simulink model "Xl_ch16_LPF_int_v5"  (Simulink 7.5)
settings: Solver=VariableStepDiscrete  StartTime=0.0  StopTime=0.001  RelTol=1e-3
values from neighbouring files (symbols this model uses):
  a2a = zeros(nFc, length(Hd.sosMatrix(:,5)))    [iirButter_SOS_init_v2.m]    (also in iirButter_SOS_init_v2_8pole.m)
  a3a = zeros(nFc, length(Hd.sosMatrix(:,6)))    [iirButter_SOS_init_v2.m]    (also in iirButter_SOS_init_v2_8pole.m)
  dt = 1/Fsim    (= 2.56e-06)    [iirButter_SOS_init_v2.m]    (also in iirButter_SOS_init_v2_8pole.m)
  Fc_min = 10    [iirButter_SOS_init_v2.m]    (also in iirButter_SOS_init_v2_8pole.m)
  ga = zeros(nFc, length(Hd.ScaleValues))    [iirButter_SOS_init_v2.m]    (also in iirButter_SOS_init_v2_8pole.m = zeros(nFc, length(Hd.ScaleValues(1:end-1))))
  rFc = (Fc_max/Fc_min)^(1/(nFc - 1))    (= 1.70532863139)    [iirButter_SOS_init_v2.m]    (also in iirButter_SOS_init_v2_8pole.m)
  Sra = 2^34|.02  |.027 |.027 |<.038| 1e-6|<2e-6|<2e-6|<2e-6|<2e-6| 8e-6|    [iirButter_SOS_init_v2.m]    (also in iirButter_SOS_init_v2_8pole.m)
  Srm = 2^34|     |     |     |     |     |     |     |     |     |  to |    [iirButter_SOS_init_v2.m]    (also in iirButter_SOS_init_v2_8pole.m)
libraries: xbsIndex_r4 x581, dspsrcs4 x16, simulink x8
(part 2 of 4)

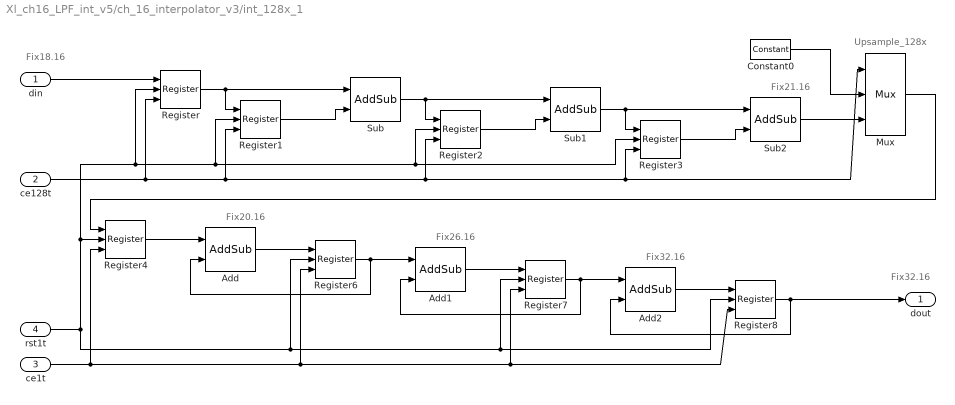
== system Xl_ch16_LPF_int_v5/ch_16_interpolator_v3/int_128x_1 ==
  note: Fix32.16
  note: Fix26.16
  note: Fix20.16
  note: Fix21.16
  note: Upsample_128x
  note: Fix32.16
  note: Fix18.16
  din : Inport
  ce128t : Inport  Port=2
  ce1t : Inport  Port=3
  rst1t : Inport  Port=4
  Add : xbsIndex_r4/AddSub  mode=Addition  use_carryin=off  use_carryout=off  en=off  latency=0  precision=User Defined  arith_type="Signed  (2's comp)"  n_bits=20  bin_pt=16  quantization=Truncate  overflow=Wrap  dbl_ovrd=off  use_behavioral_HDL=off  hw_selection=Fabric  pipelined=off  block_type=addsub
      settings: block_version=12.2
  Add1 : xbsIndex_r4/AddSub  mode=Addition  use_carryin=off  use_carryout=off  en=off  latency=0  precision=User Defined  arith_type="Signed  (2's comp)"  n_bits=26  bin_pt=16  quantization=Truncate  overflow=Wrap  dbl_ovrd=off  use_behavioral_HDL=off  hw_selection=Fabric  pipelined=off  block_type=addsub
      settings: block_version=12.2
  Add2 : xbsIndex_r4/AddSub  mode=Addition  use_carryin=off  use_carryout=off  en=off  latency=0  precision=User Defined  arith_type="Signed  (2's comp)"  n_bits=32  bin_pt=16  quantization=Truncate  overflow=Wrap  dbl_ovrd=off  use_behavioral_HDL=off  hw_selection=Fabric  pipelined=off  block_type=addsub
      settings: block_version=12.2
  Constant0 : xbsIndex_r4/Constant  arith_type=Signed (2's comp)  const=0  n_bits=21  bin_pt=16  explicit_period=off  period=1  equ=P=C  opselect=C  inp2=PCIN>>17  opr=+  inp1=P  carry=CIN  dbl_ovrd=off  block_type=constant
      settings: block_version=12.2
  Mux : xbsIndex_r4/Mux  inputs=2  en=off  latency=0  precision=Full  arith_type=Unsigned  n_bits=16  bin_pt=14  quantization=Truncate  overflow=Wrap  dbl_ovrd=off  block_type=mux
      settings: block_version=12.2
  Register{,1..4,6..8} (8 alike) : xbsIndex_r4/Register  init=0  rst=on  en=on  dbl_ovrd=off  block_type=register
      settings: block_version=12.2
  Sub : xbsIndex_r4/AddSub  mode=Subtraction  use_carryin=off  use_carryout=off  en=off  latency=0  precision=Full  arith_type=Unsigned  n_bits=16  bin_pt=14  quantization=Truncate  overflow=Wrap  dbl_ovrd=off  use_behavioral_HDL=off  hw_selection=Fabric  pipelined=off  block_type=addsub
      settings: block_version=12.2
  Sub1 : xbsIndex_r4/AddSub  mode=Subtraction  use_carryin=off  use_carryout=off  en=off  latency=0  precision=Full  arith_type=Unsigned  n_bits=16  bin_pt=14  quantization=Truncate  overflow=Wrap  dbl_ovrd=off  use_behavioral_HDL=off  hw_selection=Fabric  pipelined=off  block_type=addsub
      settings: block_version=12.2
  Sub2 : xbsIndex_r4/AddSub  mode=Subtraction  use_carryin=off  use_carryout=off  en=off  latency=0  precision=Full  arith_type=Unsigned  n_bits=16  bin_pt=14  quantization=Truncate  overflow=Wrap  dbl_ovrd=off  use_behavioral_HDL=off  hw_selection=Fabric  pipelined=off  block_type=addsub
      settings: block_version=12.2
  dout : Outport
  wires:
  rst1t/1 -> Register/2, Register1/2, Register2/2, Register3/2, Register4/2, Register6/2, Register7/2, Register8/2
  ce1t/1 -> Register4/3, Register6/3, Register8/3, Register7/3
  ce128t/1 -> Register/3, Register1/3, Mux/1, Register3/3, Register2/3
  Register8/1 -> dout/1, Add2/2
  Register7/1 -> Add2/1, Add1/2
  Register6/1 -> Add1/1, Add/2
  Constant0/1 -> Mux/2
  Add2/1 -> Register8/1
  Add1/1 -> Register7/1
  Add/1 -> Register6/1
  Register4/1 -> Add/1
  Mux/1 -> Register4/1
  din/1 -> Register/1
  Sub2/1 -> Mux/3
  Register3/1 -> Sub2/2
  Sub1/1 -> Register3/1, Sub2/1
  Register2/1 -> Sub1/2
  Sub/1 -> Register2/1, Sub1/1
  Register1/1 -> Sub/2
  Register/1 -> Register1/1, Sub/1

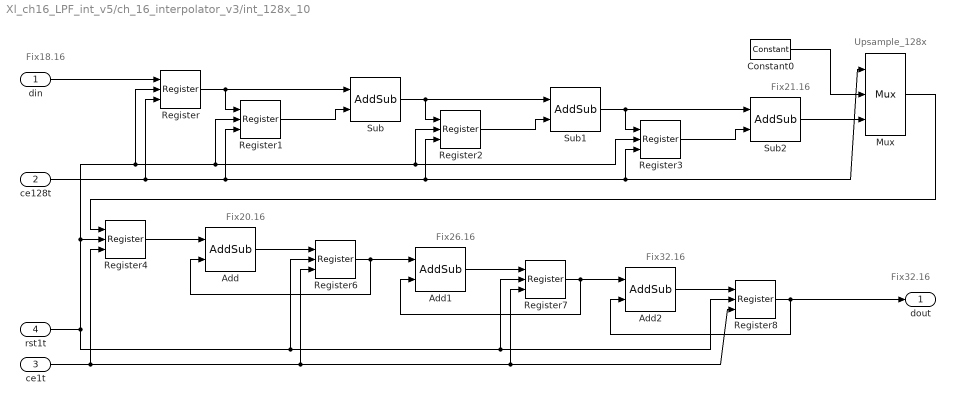
== system Xl_ch16_LPF_int_v5/ch_16_interpolator_v3/int_128x_10 ==
  note: Fix32.16
  note: Fix26.16
  note: Fix20.16
  note: Fix21.16
  note: Upsample_128x
  note: Fix32.16
  note: Fix18.16
  din : Inport
  ce128t : Inport  Port=2
  ce1t : Inport  Port=3
  rst1t : Inport  Port=4
  Add : xbsIndex_r4/AddSub  mode=Addition  use_carryin=off  use_carryout=off  en=off  latency=0  precision=User Defined  arith_type="Signed  (2's comp)"  n_bits=20  bin_pt=16  quantization=Truncate  overflow=Wrap  dbl_ovrd=off  use_behavioral_HDL=off  hw_selection=Fabric  pipelined=off  block_type=addsub
      settings: block_version=12.2
  Add1 : xbsIndex_r4/AddSub  mode=Addition  use_carryin=off  use_carryout=off  en=off  latency=0  precision=User Defined  arith_type="Signed  (2's comp)"  n_bits=26  bin_pt=16  quantization=Truncate  overflow=Wrap  dbl_ovrd=off  use_behavioral_HDL=off  hw_selection=Fabric  pipelined=off  block_type=addsub
      settings: block_version=12.2
  Add2 : xbsIndex_r4/AddSub  mode=Addition  use_carryin=off  use_carryout=off  en=off  latency=0  precision=User Defined  arith_type="Signed  (2's comp)"  n_bits=32  bin_pt=16  quantization=Truncate  overflow=Wrap  dbl_ovrd=off  use_behavioral_HDL=off  hw_selection=Fabric  pipelined=off  block_type=addsub
      settings: block_version=12.2
  Constant0 : xbsIndex_r4/Constant  arith_type=Signed (2's comp)  const=0  n_bits=21  bin_pt=16  explicit_period=off  period=1  equ=P=C  opselect=C  inp2=PCIN>>17  opr=+  inp1=P  carry=CIN  dbl_ovrd=off  block_type=constant
      settings: block_version=12.2
  Mux : xbsIndex_r4/Mux  inputs=2  en=off  latency=0  precision=Full  arith_type=Unsigned  n_bits=16  bin_pt=14  quantization=Truncate  overflow=Wrap  dbl_ovrd=off  block_type=mux
      settings: block_version=12.2
  Register{,1..4,6..8} (8 alike) : xbsIndex_r4/Register  init=0  rst=on  en=on  dbl_ovrd=off  block_type=register
      settings: block_version=12.2
  Sub : xbsIndex_r4/AddSub  mode=Subtraction  use_carryin=off  use_carryout=off  en=off  latency=0  precision=Full  arith_type=Unsigned  n_bits=16  bin_pt=14  quantization=Truncate  overflow=Wrap  dbl_ovrd=off  use_behavioral_HDL=off  hw_selection=Fabric  pipelined=off  block_type=addsub
      settings: block_version=12.2
  Sub1 : xbsIndex_r4/AddSub  mode=Subtraction  use_carryin=off  use_carryout=off  en=off  latency=0  precision=Full  arith_type=Unsigned  n_bits=16  bin_pt=14  quantization=Truncate  overflow=Wrap  dbl_ovrd=off  use_behavioral_HDL=off  hw_selection=Fabric  pipelined=off  block_type=addsub
      settings: block_version=12.2
  Sub2 : xbsIndex_r4/AddSub  mode=Subtraction  use_carryin=off  use_carryout=off  en=off  latency=0  precision=Full  arith_type=Unsigned  n_bits=16  bin_pt=14  quantization=Truncate  overflow=Wrap  dbl_ovrd=off  use_behavioral_HDL=off  hw_selection=Fabric  pipelined=off  block_type=addsub
      settings: block_version=12.2
  dout : Outport
  wires:
  rst1t/1 -> Register/2, Register1/2, Register2/2, Register3/2, Register4/2, Register6/2, Register7/2, Register8/2
  ce1t/1 -> Register4/3, Register6/3, Register8/3, Register7/3
  ce128t/1 -> Register/3, Register1/3, Mux/1, Register3/3, Register2/3
  Register8/1 -> dout/1, Add2/2
  Register7/1 -> Add2/1, Add1/2
  Register6/1 -> Add1/1, Add/2
  Constant0/1 -> Mux/2
  Add2/1 -> Register8/1
  Add1/1 -> Register7/1
  Add/1 -> Register6/1
  Register4/1 -> Add/1
  Mux/1 -> Register4/1
  din/1 -> Register/1
  Sub2/1 -> Mux/3
  Register3/1 -> Sub2/2
  Sub1/1 -> Register3/1, Sub2/1
  Register2/1 -> Sub1/2
  Sub/1 -> Register2/1, Sub1/1
  Register1/1 -> Sub/2
  Register/1 -> Register1/1, Sub/1

== system Xl_ch16_LPF_int_v5/ch_16_interpolator_v3/int_128x_11 ==
  note: Fix18.16
  note: Fix32.16
  note: Upsample_128x
  note: Fix21.16
  note: Fix20.16
  note: Fix26.16
  note: Fix32.16
  din : Inport
  ce128t : Inport  Port=2
  ce1t : Inport  Port=3
  rst1t : Inport  Port=4
  Add : xbsIndex_r4/AddSub  mode=Addition  use_carryin=off  use_carryout=off  en=off  latency=0  precision=User Defined  arith_type="Signed  (2's comp)"  n_bits=20  bin_pt=16  quantization=Truncate  overflow=Wrap  dbl_ovrd=off  use_behavioral_HDL=off  hw_selection=Fabric  pipelined=off  block_type=addsub
      settings: block_version=12.2
  Add1 : xbsIndex_r4/AddSub  mode=Addition  use_carryin=off  use_carryout=off  en=off  latency=0  precision=User Defined  arith_type="Signed  (2's comp)"  n_bits=26  bin_pt=16  quantization=Truncate  overflow=Wrap  dbl_ovrd=off  use_behavioral_HDL=off  hw_selection=Fabric  pipelined=off  block_type=addsub
      settings: block_version=12.2
  Add2 : xbsIndex_r4/AddSub  mode=Addition  use_carryin=off  use_carryout=off  en=off  latency=0  precision=User Defined  arith_type="Signed  (2's comp)"  n_bits=32  bin_pt=16  quantization=Truncate  overflow=Wrap  dbl_ovrd=off  use_behavioral_HDL=off  hw_selection=Fabric  pipelined=off  block_type=addsub
      settings: block_version=12.2
  Constant0 : xbsIndex_r4/Constant  arith_type=Signed (2's comp)  const=0  n_bits=21  bin_pt=16  explicit_period=off  period=1  equ=P=C  opselect=C  inp2=PCIN>>17  opr=+  inp1=P  carry=CIN  dbl_ovrd=off  block_type=constant
      settings: block_version=12.2
  Mux : xbsIndex_r4/Mux  inputs=2  en=off  latency=0  precision=Full  arith_type=Unsigned  n_bits=16  bin_pt=14  quantization=Truncate  overflow=Wrap  dbl_ovrd=off  block_type=mux
      settings: block_version=12.2
  Register{,1..4,6..8} (8 alike) : xbsIndex_r4/Register  init=0  rst=on  en=on  dbl_ovrd=off  block_type=register
      settings: block_version=12.2
  Sub : xbsIndex_r4/AddSub  mode=Subtraction  use_carryin=off  use_carryout=off  en=off  latency=0  precision=Full  arith_type=Unsigned  n_bits=16  bin_pt=14  quantization=Truncate  overflow=Wrap  dbl_ovrd=off  use_behavioral_HDL=off  hw_selection=Fabric  pipelined=off  block_type=addsub
      settings: block_version=12.2
  Sub1 : xbsIndex_r4/AddSub  mode=Subtraction  use_carryin=off  use_carryout=off  en=off  latency=0  precision=Full  arith_type=Unsigned  n_bits=16  bin_pt=14  quantization=Truncate  overflow=Wrap  dbl_ovrd=off  use_behavioral_HDL=off  hw_selection=Fabric  pipelined=off  block_type=addsub
      settings: block_version=12.2
  Sub2 : xbsIndex_r4/AddSub  mode=Subtraction  use_carryin=off  use_carryout=off  en=off  latency=0  precision=Full  arith_type=Unsigned  n_bits=16  bin_pt=14  quantization=Truncate  overflow=Wrap  dbl_ovrd=off  use_behavioral_HDL=off  hw_selection=Fabric  pipelined=off  block_type=addsub
      settings: block_version=12.2
  dout : Outport
  wires:
  Register/1 -> Sub/1, Register1/1
  Register1/1 -> Sub/2
  Sub/1 -> Sub1/1, Register2/1
  Register2/1 -> Sub1/2
  Sub1/1 -> Sub2/1, Register3/1
  Register3/1 -> Sub2/2
  Sub2/1 -> Mux/3
  din/1 -> Register/1
  Mux/1 -> Register4/1
  Register4/1 -> Add/1
  Add/1 -> Register6/1
  Add1/1 -> Register7/1
  Add2/1 -> Register8/1
  Constant0/1 -> Mux/2
  Register6/1 -> Add/2, Add1/1
  Register7/1 -> Add1/2, Add2/1
  Register8/1 -> Add2/2, dout/1
  ce128t/1 -> Register2/3, Register3/3, Mux/1, Register1/3, Register/3
  ce1t/1 -> Register7/3, Register8/3, Register6/3, Register4/3
  rst1t/1 -> Register8/2, Register7/2, Register6/2, Register4/2, Register3/2, Register2/2, Register1/2, Register/2

== system Xl_ch16_LPF_int_v5/ch_16_interpolator_v3/int_128x_12 ==
  note: Fix32.16
  note: Fix26.16
  note: Fix20.16
  note: Fix21.16
  note: Upsample_128x
  note: Fix32.16
  note: Fix18.16
  din : Inport
  ce128t : Inport  Port=2
  ce1t : Inport  Port=3
  rst1t : Inport  Port=4
  Add : xbsIndex_r4/AddSub  mode=Addition  use_carryin=off  use_carryout=off  en=off  latency=0  precision=User Defined  arith_type="Signed  (2's comp)"  n_bits=20  bin_pt=16  quantization=Truncate  overflow=Wrap  dbl_ovrd=off  use_behavioral_HDL=off  hw_selection=Fabric  pipelined=off  block_type=addsub
      settings: block_version=12.2
  Add1 : xbsIndex_r4/AddSub  mode=Addition  use_carryin=off  use_carryout=off  en=off  latency=0  precision=User Defined  arith_type="Signed  (2's comp)"  n_bits=26  bin_pt=16  quantization=Truncate  overflow=Wrap  dbl_ovrd=off  use_behavioral_HDL=off  hw_selection=Fabric  pipelined=off  block_type=addsub
      settings: block_version=12.2
  Add2 : xbsIndex_r4/AddSub  mode=Addition  use_carryin=off  use_carryout=off  en=off  latency=0  precision=User Defined  arith_type="Signed  (2's comp)"  n_bits=32  bin_pt=16  quantization=Truncate  overflow=Wrap  dbl_ovrd=off  use_behavioral_HDL=off  hw_selection=Fabric  pipelined=off  block_type=addsub
      settings: block_version=12.2
  Constant0 : xbsIndex_r4/Constant  arith_type=Signed (2's comp)  const=0  n_bits=21  bin_pt=16  explicit_period=off  period=1  equ=P=C  opselect=C  inp2=PCIN>>17  opr=+  inp1=P  carry=CIN  dbl_ovrd=off  block_type=constant
      settings: block_version=12.2
  Mux : xbsIndex_r4/Mux  inputs=2  en=off  latency=0  precision=Full  arith_type=Unsigned  n_bits=16  bin_pt=14  quantization=Truncate  overflow=Wrap  dbl_ovrd=off  block_type=mux
      settings: block_version=12.2
  Register{,1..4,6..8} (8 alike) : xbsIndex_r4/Register  init=0  rst=on  en=on  dbl_ovrd=off  block_type=register
      settings: block_version=12.2
  Sub : xbsIndex_r4/AddSub  mode=Subtraction  use_carryin=off  use_carryout=off  en=off  latency=0  precision=Full  arith_type=Unsigned  n_bits=16  bin_pt=14  quantization=Truncate  overflow=Wrap  dbl_ovrd=off  use_behavioral_HDL=off  hw_selection=Fabric  pipelined=off  block_type=addsub
      settings: block_version=12.2
  Sub1 : xbsIndex_r4/AddSub  mode=Subtraction  use_carryin=off  use_carryout=off  en=off  latency=0  precision=Full  arith_type=Unsigned  n_bits=16  bin_pt=14  quantization=Truncate  overflow=Wrap  dbl_ovrd=off  use_behavioral_HDL=off  hw_selection=Fabric  pipelined=off  block_type=addsub
      settings: block_version=12.2
  Sub2 : xbsIndex_r4/AddSub  mode=Subtraction  use_carryin=off  use_carryout=off  en=off  latency=0  precision=Full  arith_type=Unsigned  n_bits=16  bin_pt=14  quantization=Truncate  overflow=Wrap  dbl_ovrd=off  use_behavioral_HDL=off  hw_selection=Fabric  pipelined=off  block_type=addsub
      settings: block_version=12.2
  dout : Outport
  wires:
  rst1t/1 -> Register/2, Register1/2, Register2/2, Register3/2, Register4/2, Register6/2, Register7/2, Register8/2
  ce1t/1 -> Register4/3, Register6/3, Register8/3, Register7/3
  ce128t/1 -> Register/3, Register1/3, Mux/1, Register3/3, Register2/3
  Register8/1 -> dout/1, Add2/2
  Register7/1 -> Add2/1, Add1/2
  Register6/1 -> Add1/1, Add/2
  Constant0/1 -> Mux/2
  Add2/1 -> Register8/1
  Add1/1 -> Register7/1
  Add/1 -> Register6/1
  Register4/1 -> Add/1
  Mux/1 -> Register4/1
  din/1 -> Register/1
  Sub2/1 -> Mux/3
  Register3/1 -> Sub2/2
  Sub1/1 -> Register3/1, Sub2/1
  Register2/1 -> Sub1/2
  Sub/1 -> Register2/1, Sub1/1
  Register1/1 -> Sub/2
  Register/1 -> Register1/1, Sub/1

== system Xl_ch16_LPF_int_v5/ch_16_interpolator_v3/int_128x_13 ==
  note: Fix18.16
  note: Fix32.16
  note: Upsample_128x
  note: Fix21.16
  note: Fix20.16
  note: Fix26.16
  note: Fix32.16
  din : Inport
  ce128t : Inport  Port=2
  ce1t : Inport  Port=3
  rst1t : Inport  Port=4
  Add : xbsIndex_r4/AddSub  mode=Addition  use_carryin=off  use_carryout=off  en=off  latency=0  precision=User Defined  arith_type="Signed  (2's comp)"  n_bits=20  bin_pt=16  quantization=Truncate  overflow=Wrap  dbl_ovrd=off  use_behavioral_HDL=off  hw_selection=Fabric  pipelined=off  block_type=addsub
      settings: block_version=12.2
  Add1 : xbsIndex_r4/AddSub  mode=Addition  use_carryin=off  use_carryout=off  en=off  latency=0  precision=User Defined  arith_type="Signed  (2's comp)"  n_bits=26  bin_pt=16  quantization=Truncate  overflow=Wrap  dbl_ovrd=off  use_behavioral_HDL=off  hw_selection=Fabric  pipelined=off  block_type=addsub
      settings: block_version=12.2
  Add2 : xbsIndex_r4/AddSub  mode=Addition  use_carryin=off  use_carryout=off  en=off  latency=0  precision=User Defined  arith_type="Signed  (2's comp)"  n_bits=32  bin_pt=16  quantization=Truncate  overflow=Wrap  dbl_ovrd=off  use_behavioral_HDL=off  hw_selection=Fabric  pipelined=off  block_type=addsub
      settings: block_version=12.2
  Constant0 : xbsIndex_r4/Constant  arith_type=Signed (2's comp)  const=0  n_bits=21  bin_pt=16  explicit_period=off  period=1  equ=P=C  opselect=C  inp2=PCIN>>17  opr=+  inp1=P  carry=CIN  dbl_ovrd=off  block_type=constant
      settings: block_version=12.2
  Mux : xbsIndex_r4/Mux  inputs=2  en=off  latency=0  precision=Full  arith_type=Unsigned  n_bits=16  bin_pt=14  quantization=Truncate  overflow=Wrap  dbl_ovrd=off  block_type=mux
      settings: block_version=12.2
  Register{,1..4,6..8} (8 alike) : xbsIndex_r4/Register  init=0  rst=on  en=on  dbl_ovrd=off  block_type=register
      settings: block_version=12.2
  Sub : xbsIndex_r4/AddSub  mode=Subtraction  use_carryin=off  use_carryout=off  en=off  latency=0  precision=Full  arith_type=Unsigned  n_bits=16  bin_pt=14  quantization=Truncate  overflow=Wrap  dbl_ovrd=off  use_behavioral_HDL=off  hw_selection=Fabric  pipelined=off  block_type=addsub
      settings: block_version=12.2
  Sub1 : xbsIndex_r4/AddSub  mode=Subtraction  use_carryin=off  use_carryout=off  en=off  latency=0  precision=Full  arith_type=Unsigned  n_bits=16  bin_pt=14  quantization=Truncate  overflow=Wrap  dbl_ovrd=off  use_behavioral_HDL=off  hw_selection=Fabric  pipelined=off  block_type=addsub
      settings: block_version=12.2
  Sub2 : xbsIndex_r4/AddSub  mode=Subtraction  use_carryin=off  use_carryout=off  en=off  latency=0  precision=Full  arith_type=Unsigned  n_bits=16  bin_pt=14  quantization=Truncate  overflow=Wrap  dbl_ovrd=off  use_behavioral_HDL=off  hw_selection=Fabric  pipelined=off  block_type=addsub
      settings: block_version=12.2
  dout : Outport
  wires:
  Register/1 -> Sub/1, Register1/1
  Register1/1 -> Sub/2
  Sub/1 -> Sub1/1, Register2/1
  Register2/1 -> Sub1/2
  Sub1/1 -> Sub2/1, Register3/1
  Register3/1 -> Sub2/2
  Sub2/1 -> Mux/3
  din/1 -> Register/1
  Mux/1 -> Register4/1
  Register4/1 -> Add/1
  Add/1 -> Register6/1
  Add1/1 -> Register7/1
  Add2/1 -> Register8/1
  Constant0/1 -> Mux/2
  Register6/1 -> Add/2, Add1/1
  Register7/1 -> Add1/2, Add2/1
  Register8/1 -> Add2/2, dout/1
  ce128t/1 -> Register2/3, Register3/3, Mux/1, Register1/3, Register/3
  ce1t/1 -> Register7/3, Register8/3, Register6/3, Register4/3
  rst1t/1 -> Register8/2, Register7/2, Register6/2, Register4/2, Register3/2, Register2/2, Register1/2, Register/2

== system Xl_ch16_LPF_int_v5/ch_16_interpolator_v3/int_128x_14 ==
  note: Fix32.16
  note: Fix26.16
  note: Fix20.16
  note: Fix21.16
  note: Upsample_128x
  note: Fix32.16
  note: Fix18.16
  din : Inport
  ce128t : Inport  Port=2
  ce1t : Inport  Port=3
  rst1t : Inport  Port=4
  Add : xbsIndex_r4/AddSub  mode=Addition  use_carryin=off  use_carryout=off  en=off  latency=0  precision=User Defined  arith_type="Signed  (2's comp)"  n_bits=20  bin_pt=16  quantization=Truncate  overflow=Wrap  dbl_ovrd=off  use_behavioral_HDL=off  hw_selection=Fabric  pipelined=off  block_type=addsub
      settings: block_version=12.2
  Add1 : xbsIndex_r4/AddSub  mode=Addition  use_carryin=off  use_carryout=off  en=off  latency=0  precision=User Defined  arith_type="Signed  (2's comp)"  n_bits=26  bin_pt=16  quantization=Truncate  overflow=Wrap  dbl_ovrd=off  use_behavioral_HDL=off  hw_selection=Fabric  pipelined=off  block_type=addsub
      settings: block_version=12.2
  Add2 : xbsIndex_r4/AddSub  mode=Addition  use_carryin=off  use_carryout=off  en=off  latency=0  precision=User Defined  arith_type="Signed  (2's comp)"  n_bits=32  bin_pt=16  quantization=Truncate  overflow=Wrap  dbl_ovrd=off  use_behavioral_HDL=off  hw_selection=Fabric  pipelined=off  block_type=addsub
      settings: block_version=12.2
  Constant0 : xbsIndex_r4/Constant  arith_type=Signed (2's comp)  const=0  n_bits=21  bin_pt=16  explicit_period=off  period=1  equ=P=C  opselect=C  inp2=PCIN>>17  opr=+  inp1=P  carry=CIN  dbl_ovrd=off  block_type=constant
      settings: block_version=12.2
  Mux : xbsIndex_r4/Mux  inputs=2  en=off  latency=0  precision=Full  arith_type=Unsigned  n_bits=16  bin_pt=14  quantization=Truncate  overflow=Wrap  dbl_ovrd=off  block_type=mux
      settings: block_version=12.2
  Register{,1..4,6..8} (8 alike) : xbsIndex_r4/Register  init=0  rst=on  en=on  dbl_ovrd=off  block_type=register
      settings: block_version=12.2
  Sub : xbsIndex_r4/AddSub  mode=Subtraction  use_carryin=off  use_carryout=off  en=off  latency=0  precision=Full  arith_type=Unsigned  n_bits=16  bin_pt=14  quantization=Truncate  overflow=Wrap  dbl_ovrd=off  use_behavioral_HDL=off  hw_selection=Fabric  pipelined=off  block_type=addsub
      settings: block_version=12.2
  Sub1 : xbsIndex_r4/AddSub  mode=Subtraction  use_carryin=off  use_carryout=off  en=off  latency=0  precision=Full  arith_type=Unsigned  n_bits=16  bin_pt=14  quantization=Truncate  overflow=Wrap  dbl_ovrd=off  use_behavioral_HDL=off  hw_selection=Fabric  pipelined=off  block_type=addsub
      settings: block_version=12.2
  Sub2 : xbsIndex_r4/AddSub  mode=Subtraction  use_carryin=off  use_carryout=off  en=off  latency=0  precision=Full  arith_type=Unsigned  n_bits=16  bin_pt=14  quantization=Truncate  overflow=Wrap  dbl_ovrd=off  use_behavioral_HDL=off  hw_selection=Fabric  pipelined=off  block_type=addsub
      settings: block_version=12.2
  dout : Outport
  wires:
  rst1t/1 -> Register/2, Register1/2, Register2/2, Register3/2, Register4/2, Register6/2, Register7/2, Register8/2
  ce1t/1 -> Register4/3, Register6/3, Register8/3, Register7/3
  ce128t/1 -> Register/3, Register1/3, Mux/1, Register3/3, Register2/3
  Register8/1 -> dout/1, Add2/2
  Register7/1 -> Add2/1, Add1/2
  Register6/1 -> Add1/1, Add/2
  Constant0/1 -> Mux/2
  Add2/1 -> Register8/1
  Add1/1 -> Register7/1
  Add/1 -> Register6/1
  Register4/1 -> Add/1
  Mux/1 -> Register4/1
  din/1 -> Register/1
  Sub2/1 -> Mux/3
  Register3/1 -> Sub2/2
  Sub1/1 -> Register3/1, Sub2/1
  Register2/1 -> Sub1/2
  Sub/1 -> Register2/1, Sub1/1
  Register1/1 -> Sub/2
  Register/1 -> Register1/1, Sub/1

== system Xl_ch16_LPF_int_v5/ch_16_interpolator_v3/int_128x_15 ==
  note: Fix18.16
  note: Fix32.16
  note: Upsample_128x
  note: Fix21.16
  note: Fix20.16
  note: Fix26.16
  note: Fix32.16
  din : Inport
  ce128t : Inport  Port=2
  ce1t : Inport  Port=3
  rst1t : Inport  Port=4
  Add : xbsIndex_r4/AddSub  mode=Addition  use_carryin=off  use_carryout=off  en=off  latency=0  precision=User Defined  arith_type="Signed  (2's comp)"  n_bits=20  bin_pt=16  quantization=Truncate  overflow=Wrap  dbl_ovrd=off  use_behavioral_HDL=off  hw_selection=Fabric  pipelined=off  block_type=addsub
      settings: block_version=12.2
  Add1 : xbsIndex_r4/AddSub  mode=Addition  use_carryin=off  use_carryout=off  en=off  latency=0  precision=User Defined  arith_type="Signed  (2's comp)"  n_bits=26  bin_pt=16  quantization=Truncate  overflow=Wrap  dbl_ovrd=off  use_behavioral_HDL=off  hw_selection=Fabric  pipelined=off  block_type=addsub
      settings: block_version=12.2
  Add2 : xbsIndex_r4/AddSub  mode=Addition  use_carryin=off  use_carryout=off  en=off  latency=0  precision=User Defined  arith_type="Signed  (2's comp)"  n_bits=32  bin_pt=16  quantization=Truncate  overflow=Wrap  dbl_ovrd=off  use_behavioral_HDL=off  hw_selection=Fabric  pipelined=off  block_type=addsub
      settings: block_version=12.2
  Constant0 : xbsIndex_r4/Constant  arith_type=Signed (2's comp)  const=0  n_bits=21  bin_pt=16  explicit_period=off  period=1  equ=P=C  opselect=C  inp2=PCIN>>17  opr=+  inp1=P  carry=CIN  dbl_ovrd=off  block_type=constant
      settings: block_version=12.2
  Mux : xbsIndex_r4/Mux  inputs=2  en=off  latency=0  precision=Full  arith_type=Unsigned  n_bits=16  bin_pt=14  quantization=Truncate  overflow=Wrap  dbl_ovrd=off  block_type=mux
      settings: block_version=12.2
  Register{,1..4,6..8} (8 alike) : xbsIndex_r4/Register  init=0  rst=on  en=on  dbl_ovrd=off  block_type=register
      settings: block_version=12.2
  Sub : xbsIndex_r4/AddSub  mode=Subtraction  use_carryin=off  use_carryout=off  en=off  latency=0  precision=Full  arith_type=Unsigned  n_bits=16  bin_pt=14  quantization=Truncate  overflow=Wrap  dbl_ovrd=off  use_behavioral_HDL=off  hw_selection=Fabric  pipelined=off  block_type=addsub
      settings: block_version=12.2
  Sub1 : xbsIndex_r4/AddSub  mode=Subtraction  use_carryin=off  use_carryout=off  en=off  latency=0  precision=Full  arith_type=Unsigned  n_bits=16  bin_pt=14  quantization=Truncate  overflow=Wrap  dbl_ovrd=off  use_behavioral_HDL=off  hw_selection=Fabric  pipelined=off  block_type=addsub
      settings: block_version=12.2
  Sub2 : xbsIndex_r4/AddSub  mode=Subtraction  use_carryin=off  use_carryout=off  en=off  latency=0  precision=Full  arith_type=Unsigned  n_bits=16  bin_pt=14  quantization=Truncate  overflow=Wrap  dbl_ovrd=off  use_behavioral_HDL=off  hw_selection=Fabric  pipelined=off  block_type=addsub
      settings: block_version=12.2
  dout : Outport
  wires:
  Register/1 -> Sub/1, Register1/1
  Register1/1 -> Sub/2
  Sub/1 -> Sub1/1, Register2/1
  Register2/1 -> Sub1/2
  Sub1/1 -> Sub2/1, Register3/1
  Register3/1 -> Sub2/2
  Sub2/1 -> Mux/3
  din/1 -> Register/1
  Mux/1 -> Register4/1
  Register4/1 -> Add/1
  Add/1 -> Register6/1
  Add1/1 -> Register7/1
  Add2/1 -> Register8/1
  Constant0/1 -> Mux/2
  Register6/1 -> Add/2, Add1/1
  Register7/1 -> Add1/2, Add2/1
  Register8/1 -> Add2/2, dout/1
  ce128t/1 -> Register2/3, Register3/3, Mux/1, Register1/3, Register/3
  ce1t/1 -> Register7/3, Register8/3, Register6/3, Register4/3
  rst1t/1 -> Register8/2, Register7/2, Register6/2, Register4/2, Register3/2, Register2/2, Register1/2, Register/2

== system Xl_ch16_LPF_int_v5/ch_16_interpolator_v3/int_128x_16 ==
  note: Fix32.16
  note: Fix26.16
  note: Fix20.16
  note: Fix21.16
  note: Upsample_128x
  note: Fix32.16
  note: Fix18.16
  din : Inport
  ce128t : Inport  Port=2
  ce1t : Inport  Port=3
  rst1t : Inport  Port=4
  Add : xbsIndex_r4/AddSub  mode=Addition  use_carryin=off  use_carryout=off  en=off  latency=0  precision=User Defined  arith_type="Signed  (2's comp)"  n_bits=20  bin_pt=16  quantization=Truncate  overflow=Wrap  dbl_ovrd=off  use_behavioral_HDL=off  hw_selection=Fabric  pipelined=off  block_type=addsub
      settings: block_version=12.2
  Add1 : xbsIndex_r4/AddSub  mode=Addition  use_carryin=off  use_carryout=off  en=off  latency=0  precision=User Defined  arith_type="Signed  (2's comp)"  n_bits=26  bin_pt=16  quantization=Truncate  overflow=Wrap  dbl_ovrd=off  use_behavioral_HDL=off  hw_selection=Fabric  pipelined=off  block_type=addsub
      settings: block_version=12.2
  Add2 : xbsIndex_r4/AddSub  mode=Addition  use_carryin=off  use_carryout=off  en=off  latency=0  precision=User Defined  arith_type="Signed  (2's comp)"  n_bits=32  bin_pt=16  quantization=Truncate  overflow=Wrap  dbl_ovrd=off  use_behavioral_HDL=off  hw_selection=Fabric  pipelined=off  block_type=addsub
      settings: block_version=12.2
  Constant0 : xbsIndex_r4/Constant  arith_type=Signed (2's comp)  const=0  n_bits=21  bin_pt=16  explicit_period=off  period=1  equ=P=C  opselect=C  inp2=PCIN>>17  opr=+  inp1=P  carry=CIN  dbl_ovrd=off  block_type=constant
      settings: block_version=12.2
  Mux : xbsIndex_r4/Mux  inputs=2  en=off  latency=0  precision=Full  arith_type=Unsigned  n_bits=16  bin_pt=14  quantization=Truncate  overflow=Wrap  dbl_ovrd=off  block_type=mux
      settings: block_version=12.2
  Register{,1..4,6..8} (8 alike) : xbsIndex_r4/Register  init=0  rst=on  en=on  dbl_ovrd=off  block_type=register
      settings: block_version=12.2
  Sub : xbsIndex_r4/AddSub  mode=Subtraction  use_carryin=off  use_carryout=off  en=off  latency=0  precision=Full  arith_type=Unsigned  n_bits=16  bin_pt=14  quantization=Truncate  overflow=Wrap  dbl_ovrd=off  use_behavioral_HDL=off  hw_selection=Fabric  pipelined=off  block_type=addsub
      settings: block_version=12.2
  Sub1 : xbsIndex_r4/AddSub  mode=Subtraction  use_carryin=off  use_carryout=off  en=off  latency=0  precision=Full  arith_type=Unsigned  n_bits=16  bin_pt=14  quantization=Truncate  overflow=Wrap  dbl_ovrd=off  use_behavioral_HDL=off  hw_selection=Fabric  pipelined=off  block_type=addsub
      settings: block_version=12.2
  Sub2 : xbsIndex_r4/AddSub  mode=Subtraction  use_carryin=off  use_carryout=off  en=off  latency=0  precision=Full  arith_type=Unsigned  n_bits=16  bin_pt=14  quantization=Truncate  overflow=Wrap  dbl_ovrd=off  use_behavioral_HDL=off  hw_selection=Fabric  pipelined=off  block_type=addsub
      settings: block_version=12.2
  dout : Outport
  wires:
  rst1t/1 -> Register/2, Register1/2, Register2/2, Register3/2, Register4/2, Register6/2, Register7/2, Register8/2
  ce1t/1 -> Register4/3, Register6/3, Register8/3, Register7/3
  ce128t/1 -> Register/3, Register1/3, Mux/1, Register3/3, Register2/3
  Register8/1 -> dout/1, Add2/2
  Register7/1 -> Add2/1, Add1/2
  Register6/1 -> Add1/1, Add/2
  Constant0/1 -> Mux/2
  Add2/1 -> Register8/1
  Add1/1 -> Register7/1
  Add/1 -> Register6/1
  Register4/1 -> Add/1
  Mux/1 -> Register4/1
  din/1 -> Register/1
  Sub2/1 -> Mux/3
  Register3/1 -> Sub2/2
  Sub1/1 -> Register3/1, Sub2/1
  Register2/1 -> Sub1/2
  Sub/1 -> Register2/1, Sub1/1
  Register1/1 -> Sub/2
  Register/1 -> Register1/1, Sub/1

== system Xl_ch16_LPF_int_v5/ch_16_interpolator_v3/int_128x_2 ==
  note: Fix18.16
  note: Fix32.16
  note: Upsample_128x
  note: Fix21.16
  note: Fix20.16
  note: Fix26.16
  note: Fix32.16
  din : Inport
  ce128t : Inport  Port=2
  ce1t : Inport  Port=3
  rst1t : Inport  Port=4
  Add : xbsIndex_r4/AddSub  mode=Addition  use_carryin=off  use_carryout=off  en=off  latency=0  precision=User Defined  arith_type="Signed  (2's comp)"  n_bits=20  bin_pt=16  quantization=Truncate  overflow=Wrap  dbl_ovrd=off  use_behavioral_HDL=off  hw_selection=Fabric  pipelined=off  block_type=addsub
      settings: block_version=12.2
  Add1 : xbsIndex_r4/AddSub  mode=Addition  use_carryin=off  use_carryout=off  en=off  latency=0  precision=User Defined  arith_type="Signed  (2's comp)"  n_bits=26  bin_pt=16  quantization=Truncate  overflow=Wrap  dbl_ovrd=off  use_behavioral_HDL=off  hw_selection=Fabric  pipelined=off  block_type=addsub
      settings: block_version=12.2
  Add2 : xbsIndex_r4/AddSub  mode=Addition  use_carryin=off  use_carryout=off  en=off  latency=0  precision=User Defined  arith_type="Signed  (2's comp)"  n_bits=32  bin_pt=16  quantization=Truncate  overflow=Wrap  dbl_ovrd=off  use_behavioral_HDL=off  hw_selection=Fabric  pipelined=off  block_type=addsub
      settings: block_version=12.2
  Constant0 : xbsIndex_r4/Constant  arith_type=Signed (2's comp)  const=0  n_bits=21  bin_pt=16  explicit_period=off  period=1  equ=P=C  opselect=C  inp2=PCIN>>17  opr=+  inp1=P  carry=CIN  dbl_ovrd=off  block_type=constant
      settings: block_version=12.2
  Mux : xbsIndex_r4/Mux  inputs=2  en=off  latency=0  precision=Full  arith_type=Unsigned  n_bits=16  bin_pt=14  quantization=Truncate  overflow=Wrap  dbl_ovrd=off  block_type=mux
      settings: block_version=12.2
  Register{,1..4,6..8} (8 alike) : xbsIndex_r4/Register  init=0  rst=on  en=on  dbl_ovrd=off  block_type=register
      settings: block_version=12.2
  Sub : xbsIndex_r4/AddSub  mode=Subtraction  use_carryin=off  use_carryout=off  en=off  latency=0  precision=Full  arith_type=Unsigned  n_bits=16  bin_pt=14  quantization=Truncate  overflow=Wrap  dbl_ovrd=off  use_behavioral_HDL=off  hw_selection=Fabric  pipelined=off  block_type=addsub
      settings: block_version=12.2
  Sub1 : xbsIndex_r4/AddSub  mode=Subtraction  use_carryin=off  use_carryout=off  en=off  latency=0  precision=Full  arith_type=Unsigned  n_bits=16  bin_pt=14  quantization=Truncate  overflow=Wrap  dbl_ovrd=off  use_behavioral_HDL=off  hw_selection=Fabric  pipelined=off  block_type=addsub
      settings: block_version=12.2
  Sub2 : xbsIndex_r4/AddSub  mode=Subtraction  use_carryin=off  use_carryout=off  en=off  latency=0  precision=Full  arith_type=Unsigned  n_bits=16  bin_pt=14  quantization=Truncate  overflow=Wrap  dbl_ovrd=off  use_behavioral_HDL=off  hw_selection=Fabric  pipelined=off  block_type=addsub
      settings: block_version=12.2
  dout : Outport
  wires:
  Register/1 -> Sub/1, Register1/1
  Register1/1 -> Sub/2
  Sub/1 -> Sub1/1, Register2/1
  Register2/1 -> Sub1/2
  Sub1/1 -> Sub2/1, Register3/1
  Register3/1 -> Sub2/2
  Sub2/1 -> Mux/3
  din/1 -> Register/1
  Mux/1 -> Register4/1
  Register4/1 -> Add/1
  Add/1 -> Register6/1
  Add1/1 -> Register7/1
  Add2/1 -> Register8/1
  Constant0/1 -> Mux/2
  Register6/1 -> Add/2, Add1/1
  Register7/1 -> Add1/2, Add2/1
  Register8/1 -> Add2/2, dout/1
  ce128t/1 -> Register2/3, Register3/3, Mux/1, Register1/3, Register/3
  ce1t/1 -> Register7/3, Register8/3, Register6/3, Register4/3
  rst1t/1 -> Register8/2, Register7/2, Register6/2, Register4/2, Register3/2, Register2/2, Register1/2, Register/2

== system Xl_ch16_LPF_int_v5/ch_16_interpolator_v3/int_128x_3 ==
  note: Fix32.16
  note: Fix26.16
  note: Fix20.16
  note: Fix21.16
  note: Upsample_128x
  note: Fix32.16
  note: Fix18.16
  din : Inport
  ce128t : Inport  Port=2
  ce1t : Inport  Port=3
  rst1t : Inport  Port=4
  Add : xbsIndex_r4/AddSub  mode=Addition  use_carryin=off  use_carryout=off  en=off  latency=0  precision=User Defined  arith_type="Signed  (2's comp)"  n_bits=20  bin_pt=16  quantization=Truncate  overflow=Wrap  dbl_ovrd=off  use_behavioral_HDL=off  hw_selection=Fabric  pipelined=off  block_type=addsub
      settings: block_version=12.2
  Add1 : xbsIndex_r4/AddSub  mode=Addition  use_carryin=off  use_carryout=off  en=off  latency=0  precision=User Defined  arith_type="Signed  (2's comp)"  n_bits=26  bin_pt=16  quantization=Truncate  overflow=Wrap  dbl_ovrd=off  use_behavioral_HDL=off  hw_selection=Fabric  pipelined=off  block_type=addsub
      settings: block_version=12.2
  Add2 : xbsIndex_r4/AddSub  mode=Addition  use_carryin=off  use_carryout=off  en=off  latency=0  precision=User Defined  arith_type="Signed  (2's comp)"  n_bits=32  bin_pt=16  quantization=Truncate  overflow=Wrap  dbl_ovrd=off  use_behavioral_HDL=off  hw_selection=Fabric  pipelined=off  block_type=addsub
      settings: block_version=12.2
  Constant0 : xbsIndex_r4/Constant  arith_type=Signed (2's comp)  const=0  n_bits=21  bin_pt=16  explicit_period=off  period=1  equ=P=C  opselect=C  inp2=PCIN>>17  opr=+  inp1=P  carry=CIN  dbl_ovrd=off  block_type=constant
      settings: block_version=12.2
  Mux : xbsIndex_r4/Mux  inputs=2  en=off  latency=0  precision=Full  arith_type=Unsigned  n_bits=16  bin_pt=14  quantization=Truncate  overflow=Wrap  dbl_ovrd=off  block_type=mux
      settings: block_version=12.2
  Register{,1..4,6..8} (8 alike) : xbsIndex_r4/Register  init=0  rst=on  en=on  dbl_ovrd=off  block_type=register
      settings: block_version=12.2
  Sub : xbsIndex_r4/AddSub  mode=Subtraction  use_carryin=off  use_carryout=off  en=off  latency=0  precision=Full  arith_type=Unsigned  n_bits=16  bin_pt=14  quantization=Truncate  overflow=Wrap  dbl_ovrd=off  use_behavioral_HDL=off  hw_selection=Fabric  pipelined=off  block_type=addsub
      settings: block_version=12.2
  Sub1 : xbsIndex_r4/AddSub  mode=Subtraction  use_carryin=off  use_carryout=off  en=off  latency=0  precision=Full  arith_type=Unsigned  n_bits=16  bin_pt=14  quantization=Truncate  overflow=Wrap  dbl_ovrd=off  use_behavioral_HDL=off  hw_selection=Fabric  pipelined=off  block_type=addsub
      settings: block_version=12.2
  Sub2 : xbsIndex_r4/AddSub  mode=Subtraction  use_carryin=off  use_carryout=off  en=off  latency=0  precision=Full  arith_type=Unsigned  n_bits=16  bin_pt=14  quantization=Truncate  overflow=Wrap  dbl_ovrd=off  use_behavioral_HDL=off  hw_selection=Fabric  pipelined=off  block_type=addsub
      settings: block_version=12.2
  dout : Outport
  wires:
  rst1t/1 -> Register/2, Register1/2, Register2/2, Register3/2, Register4/2, Register6/2, Register7/2, Register8/2
  ce1t/1 -> Register4/3, Register6/3, Register8/3, Register7/3
  ce128t/1 -> Register/3, Register1/3, Mux/1, Register3/3, Register2/3
  Register8/1 -> dout/1, Add2/2
  Register7/1 -> Add2/1, Add1/2
  Register6/1 -> Add1/1, Add/2
  Constant0/1 -> Mux/2
  Add2/1 -> Register8/1
  Add1/1 -> Register7/1
  Add/1 -> Register6/1
  Register4/1 -> Add/1
  Mux/1 -> Register4/1
  din/1 -> Register/1
  Sub2/1 -> Mux/3
  Register3/1 -> Sub2/2
  Sub1/1 -> Register3/1, Sub2/1
  Register2/1 -> Sub1/2
  Sub/1 -> Register2/1, Sub1/1
  Register1/1 -> Sub/2
  Register/1 -> Register1/1, Sub/1

== system Xl_ch16_LPF_int_v5/ch_16_interpolator_v3/int_128x_4 ==
  note: Fix18.16
  note: Fix32.16
  note: Upsample_128x
  note: Fix21.16
  note: Fix20.16
  note: Fix26.16
  note: Fix32.16
  din : Inport
  ce128t : Inport  Port=2
  ce1t : Inport  Port=3
  rst1t : Inport  Port=4
  Add : xbsIndex_r4/AddSub  mode=Addition  use_carryin=off  use_carryout=off  en=off  latency=0  precision=User Defined  arith_type="Signed  (2's comp)"  n_bits=20  bin_pt=16  quantization=Truncate  overflow=Wrap  dbl_ovrd=off  use_behavioral_HDL=off  hw_selection=Fabric  pipelined=off  block_type=addsub
      settings: block_version=12.2
  Add1 : xbsIndex_r4/AddSub  mode=Addition  use_carryin=off  use_carryout=off  en=off  latency=0  precision=User Defined  arith_type="Signed  (2's comp)"  n_bits=26  bin_pt=16  quantization=Truncate  overflow=Wrap  dbl_ovrd=off  use_behavioral_HDL=off  hw_selection=Fabric  pipelined=off  block_type=addsub
      settings: block_version=12.2
  Add2 : xbsIndex_r4/AddSub  mode=Addition  use_carryin=off  use_carryout=off  en=off  latency=0  precision=User Defined  arith_type="Signed  (2's comp)"  n_bits=32  bin_pt=16  quantization=Truncate  overflow=Wrap  dbl_ovrd=off  use_behavioral_HDL=off  hw_selection=Fabric  pipelined=off  block_type=addsub
      settings: block_version=12.2
  Constant0 : xbsIndex_r4/Constant  arith_type=Signed (2's comp)  const=0  n_bits=21  bin_pt=16  explicit_period=off  period=1  equ=P=C  opselect=C  inp2=PCIN>>17  opr=+  inp1=P  carry=CIN  dbl_ovrd=off  block_type=constant
      settings: block_version=12.2
  Mux : xbsIndex_r4/Mux  inputs=2  en=off  latency=0  precision=Full  arith_type=Unsigned  n_bits=16  bin_pt=14  quantization=Truncate  overflow=Wrap  dbl_ovrd=off  block_type=mux
      settings: block_version=12.2
  Register{,1..4,6..8} (8 alike) : xbsIndex_r4/Register  init=0  rst=on  en=on  dbl_ovrd=off  block_type=register
      settings: block_version=12.2
  Sub : xbsIndex_r4/AddSub  mode=Subtraction  use_carryin=off  use_carryout=off  en=off  latency=0  precision=Full  arith_type=Unsigned  n_bits=16  bin_pt=14  quantization=Truncate  overflow=Wrap  dbl_ovrd=off  use_behavioral_HDL=off  hw_selection=Fabric  pipelined=off  block_type=addsub
      settings: block_version=12.2
  Sub1 : xbsIndex_r4/AddSub  mode=Subtraction  use_carryin=off  use_carryout=off  en=off  latency=0  precision=Full  arith_type=Unsigned  n_bits=16  bin_pt=14  quantization=Truncate  overflow=Wrap  dbl_ovrd=off  use_behavioral_HDL=off  hw_selection=Fabric  pipelined=off  block_type=addsub
      settings: block_version=12.2
  Sub2 : xbsIndex_r4/AddSub  mode=Subtraction  use_carryin=off  use_carryout=off  en=off  latency=0  precision=Full  arith_type=Unsigned  n_bits=16  bin_pt=14  quantization=Truncate  overflow=Wrap  dbl_ovrd=off  use_behavioral_HDL=off  hw_selection=Fabric  pipelined=off  block_type=addsub
      settings: block_version=12.2
  dout : Outport
  wires:
  Register/1 -> Sub/1, Register1/1
  Register1/1 -> Sub/2
  Sub/1 -> Sub1/1, Register2/1
  Register2/1 -> Sub1/2
  Sub1/1 -> Sub2/1, Register3/1
  Register3/1 -> Sub2/2
  Sub2/1 -> Mux/3
  din/1 -> Register/1
  Mux/1 -> Register4/1
  Register4/1 -> Add/1
  Add/1 -> Register6/1
  Add1/1 -> Register7/1
  Add2/1 -> Register8/1
  Constant0/1 -> Mux/2
  Register6/1 -> Add/2, Add1/1
  Register7/1 -> Add1/2, Add2/1
  Register8/1 -> Add2/2, dout/1
  ce128t/1 -> Register2/3, Register3/3, Mux/1, Register1/3, Register/3
  ce1t/1 -> Register7/3, Register8/3, Register6/3, Register4/3
  rst1t/1 -> Register8/2, Register7/2, Register6/2, Register4/2, Register3/2, Register2/2, Register1/2, Register/2

== system Xl_ch16_LPF_int_v5/ch_16_interpolator_v3/int_128x_5 ==
  note: Fix32.16
  note: Fix26.16
  note: Fix20.16
  note: Fix21.16
  note: Upsample_128x
  note: Fix32.16
  note: Fix18.16
  din : Inport
  ce128t : Inport  Port=2
  ce1t : Inport  Port=3
  rst1t : Inport  Port=4
  Add : xbsIndex_r4/AddSub  mode=Addition  use_carryin=off  use_carryout=off  en=off  latency=0  precision=User Defined  arith_type="Signed  (2's comp)"  n_bits=20  bin_pt=16  quantization=Truncate  overflow=Wrap  dbl_ovrd=off  use_behavioral_HDL=off  hw_selection=Fabric  pipelined=off  block_type=addsub
      settings: block_version=12.2
  Add1 : xbsIndex_r4/AddSub  mode=Addition  use_carryin=off  use_carryout=off  en=off  latency=0  precision=User Defined  arith_type="Signed  (2's comp)"  n_bits=26  bin_pt=16  quantization=Truncate  overflow=Wrap  dbl_ovrd=off  use_behavioral_HDL=off  hw_selection=Fabric  pipelined=off  block_type=addsub
      settings: block_version=12.2
  Add2 : xbsIndex_r4/AddSub  mode=Addition  use_carryin=off  use_carryout=off  en=off  latency=0  precision=User Defined  arith_type="Signed  (2's comp)"  n_bits=32  bin_pt=16  quantization=Truncate  overflow=Wrap  dbl_ovrd=off  use_behavioral_HDL=off  hw_selection=Fabric  pipelined=off  block_type=addsub
      settings: block_version=12.2
  Constant0 : xbsIndex_r4/Constant  arith_type=Signed (2's comp)  const=0  n_bits=21  bin_pt=16  explicit_period=off  period=1  equ=P=C  opselect=C  inp2=PCIN>>17  opr=+  inp1=P  carry=CIN  dbl_ovrd=off  block_type=constant
      settings: block_version=12.2
  Mux : xbsIndex_r4/Mux  inputs=2  en=off  latency=0  precision=Full  arith_type=Unsigned  n_bits=16  bin_pt=14  quantization=Truncate  overflow=Wrap  dbl_ovrd=off  block_type=mux
      settings: block_version=12.2
  Register{,1..4,6..8} (8 alike) : xbsIndex_r4/Register  init=0  rst=on  en=on  dbl_ovrd=off  block_type=register
      settings: block_version=12.2
  Sub : xbsIndex_r4/AddSub  mode=Subtraction  use_carryin=off  use_carryout=off  en=off  latency=0  precision=Full  arith_type=Unsigned  n_bits=16  bin_pt=14  quantization=Truncate  overflow=Wrap  dbl_ovrd=off  use_behavioral_HDL=off  hw_selection=Fabric  pipelined=off  block_type=addsub
      settings: block_version=12.2
  Sub1 : xbsIndex_r4/AddSub  mode=Subtraction  use_carryin=off  use_carryout=off  en=off  latency=0  precision=Full  arith_type=Unsigned  n_bits=16  bin_pt=14  quantization=Truncate  overflow=Wrap  dbl_ovrd=off  use_behavioral_HDL=off  hw_selection=Fabric  pipelined=off  block_type=addsub
      settings: block_version=12.2
  Sub2 : xbsIndex_r4/AddSub  mode=Subtraction  use_carryin=off  use_carryout=off  en=off  latency=0  precision=Full  arith_type=Unsigned  n_bits=16  bin_pt=14  quantization=Truncate  overflow=Wrap  dbl_ovrd=off  use_behavioral_HDL=off  hw_selection=Fabric  pipelined=off  block_type=addsub
      settings: block_version=12.2
  dout : Outport
  wires:
  rst1t/1 -> Register/2, Register1/2, Register2/2, Register3/2, Register4/2, Register6/2, Register7/2, Register8/2
  ce1t/1 -> Register4/3, Register6/3, Register8/3, Register7/3
  ce128t/1 -> Register/3, Register1/3, Mux/1, Register3/3, Register2/3
  Register8/1 -> dout/1, Add2/2
  Register7/1 -> Add2/1, Add1/2
  Register6/1 -> Add1/1, Add/2
  Constant0/1 -> Mux/2
  Add2/1 -> Register8/1
  Add1/1 -> Register7/1
  Add/1 -> Register6/1
  Register4/1 -> Add/1
  Mux/1 -> Register4/1
  din/1 -> Register/1
  Sub2/1 -> Mux/3
  Register3/1 -> Sub2/2
  Sub1/1 -> Register3/1, Sub2/1
  Register2/1 -> Sub1/2
  Sub/1 -> Register2/1, Sub1/1
  Register1/1 -> Sub/2
  Register/1 -> Register1/1, Sub/1

== system Xl_ch16_LPF_int_v5/ch_16_interpolator_v3/int_128x_6 ==
  note: Fix18.16
  note: Fix32.16
  note: Upsample_128x
  note: Fix21.16
  note: Fix20.16
  note: Fix26.16
  note: Fix32.16
  din : Inport
  ce128t : Inport  Port=2
  ce1t : Inport  Port=3
  rst1t : Inport  Port=4
  Add : xbsIndex_r4/AddSub  mode=Addition  use_carryin=off  use_carryout=off  en=off  latency=0  precision=User Defined  arith_type="Signed  (2's comp)"  n_bits=20  bin_pt=16  quantization=Truncate  overflow=Wrap  dbl_ovrd=off  use_behavioral_HDL=off  hw_selection=Fabric  pipelined=off  block_type=addsub
      settings: block_version=12.2
  Add1 : xbsIndex_r4/AddSub  mode=Addition  use_carryin=off  use_carryout=off  en=off  latency=0  precision=User Defined  arith_type="Signed  (2's comp)"  n_bits=26  bin_pt=16  quantization=Truncate  overflow=Wrap  dbl_ovrd=off  use_behavioral_HDL=off  hw_selection=Fabric  pipelined=off  block_type=addsub
      settings: block_version=12.2
  Add2 : xbsIndex_r4/AddSub  mode=Addition  use_carryin=off  use_carryout=off  en=off  latency=0  precision=User Defined  arith_type="Signed  (2's comp)"  n_bits=32  bin_pt=16  quantization=Truncate  overflow=Wrap  dbl_ovrd=off  use_behavioral_HDL=off  hw_selection=Fabric  pipelined=off  block_type=addsub
      settings: block_version=12.2
  Constant0 : xbsIndex_r4/Constant  arith_type=Signed (2's comp)  const=0  n_bits=21  bin_pt=16  explicit_period=off  period=1  equ=P=C  opselect=C  inp2=PCIN>>17  opr=+  inp1=P  carry=CIN  dbl_ovrd=off  block_type=constant
      settings: block_version=12.2
  Mux : xbsIndex_r4/Mux  inputs=2  en=off  latency=0  precision=Full  arith_type=Unsigned  n_bits=16  bin_pt=14  quantization=Truncate  overflow=Wrap  dbl_ovrd=off  block_type=mux
      settings: block_version=12.2
  Register{,1..4,6..8} (8 alike) : xbsIndex_r4/Register  init=0  rst=on  en=on  dbl_ovrd=off  block_type=register
      settings: block_version=12.2
  Sub : xbsIndex_r4/AddSub  mode=Subtraction  use_carryin=off  use_carryout=off  en=off  latency=0  precision=Full  arith_type=Unsigned  n_bits=16  bin_pt=14  quantization=Truncate  overflow=Wrap  dbl_ovrd=off  use_behavioral_HDL=off  hw_selection=Fabric  pipelined=off  block_type=addsub
      settings: block_version=12.2
  Sub1 : xbsIndex_r4/AddSub  mode=Subtraction  use_carryin=off  use_carryout=off  en=off  latency=0  precision=Full  arith_type=Unsigned  n_bits=16  bin_pt=14  quantization=Truncate  overflow=Wrap  dbl_ovrd=off  use_behavioral_HDL=off  hw_selection=Fabric  pipelined=off  block_type=addsub
      settings: block_version=12.2
  Sub2 : xbsIndex_r4/AddSub  mode=Subtraction  use_carryin=off  use_carryout=off  en=off  latency=0  precision=Full  arith_type=Unsigned  n_bits=16  bin_pt=14  quantization=Truncate  overflow=Wrap  dbl_ovrd=off  use_behavioral_HDL=off  hw_selection=Fabric  pipelined=off  block_type=addsub
      settings: block_version=12.2
  dout : Outport
  wires:
  Register/1 -> Sub/1, Register1/1
  Register1/1 -> Sub/2
  Sub/1 -> Sub1/1, Register2/1
  Register2/1 -> Sub1/2
  Sub1/1 -> Sub2/1, Register3/1
  Register3/1 -> Sub2/2
  Sub2/1 -> Mux/3
  din/1 -> Register/1
  Mux/1 -> Register4/1
  Register4/1 -> Add/1
  Add/1 -> Register6/1
  Add1/1 -> Register7/1
  Add2/1 -> Register8/1
  Constant0/1 -> Mux/2
  Register6/1 -> Add/2, Add1/1
  Register7/1 -> Add1/2, Add2/1
  Register8/1 -> Add2/2, dout/1
  ce128t/1 -> Register2/3, Register3/3, Mux/1, Register1/3, Register/3
  ce1t/1 -> Register7/3, Register8/3, Register6/3, Register4/3
  rst1t/1 -> Register8/2, Register7/2, Register6/2, Register4/2, Register3/2, Register2/2, Register1/2, Register/2
